simulink model "sist_1_ord_stabile"  (R2024b)
settings: Solver=VariableStepAuto  StartTime=0.0  StopTime=10.0  RelTol=1e-3
libraries: simulink x1

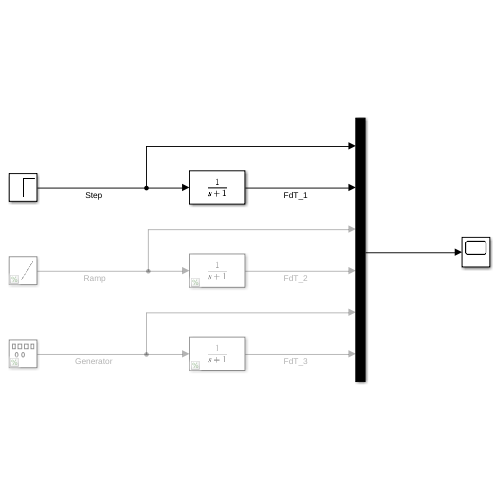
[thumbnail: Simulink's stored preview of the top-level diagram]
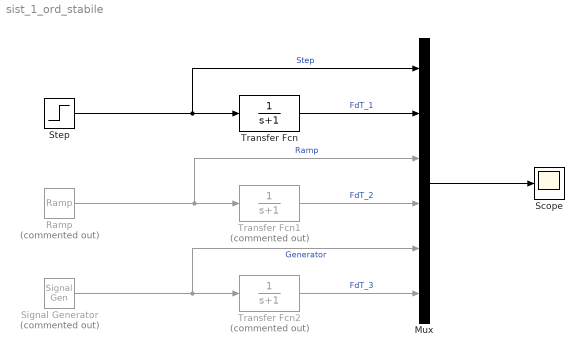
== system sist_1_ord_stabile ==
  Mux : Mux  Inputs=6
  Ramp : simulink/Sources/Ramp  Commented=on  slope=1  start=0  InitialOutput=0
  Scope : Scope
  Signal Generator : SignalGenerator  Commented=on  WaveForm=square  Units=rad/sec
  Step : Step  SampleTime=0
  Transfer Fcn : TransferFcn  Denominator=[1 1]
  Transfer Fcn1 : TransferFcn  Commented=on  Denominator=[1 1]
  Transfer Fcn2 : TransferFcn  Commented=on  Denominator=[1 1]
  wires:
  Step/1 -> Mux/1, Transfer Fcn/1  "Step"
  Ramp/1 -> Mux/3, Transfer Fcn1/1  "Ramp"
  Signal Generator/1 -> Mux/5, Transfer Fcn2/1  "Generator"
  Transfer Fcn/1 -> Mux/2  "FdT_1"
  Transfer Fcn1/1 -> Mux/4  "FdT_2"
  Transfer Fcn2/1 -> Mux/6  "FdT_3"
  Mux/1 -> Scope/1
